simulink model "SMC"  (R2018a)
settings: Solver=FixedStepAuto  StartTime=0.0  StopTime=tsim  FixedStep=ts  RelTol=1e-3
values from neighbouring files (symbols this model uses):
  m = 1    [SMCstart.m]
settings Model: Creator=Chi  LastModifiedBy=Chi

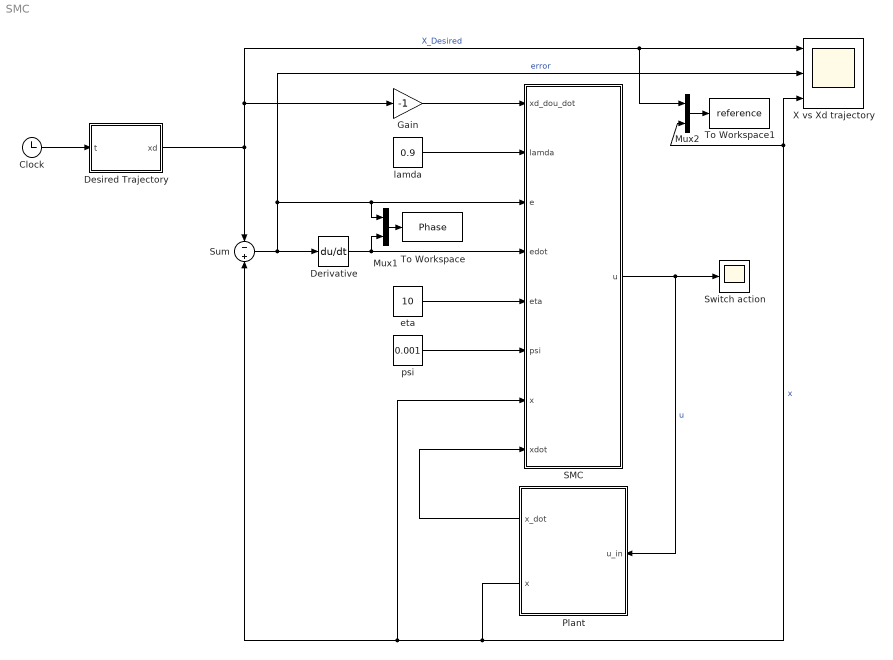
== system SMC ==
  Clock : Clock
  Derivative : Derivative
  Desired Trajectory : MATLAB Function  TreatAsAtomicUnit=on
  Gain : Gain  Gain=-1
  Mux1 : Mux  Inputs=2
  Mux2 : Mux  Inputs=2
  Plant : Subsystem
  SMC : MATLAB Function  TreatAsAtomicUnit=on
  Sum : Sum  Inputs=-+
  Switch action : Scope
  To Workspace : ToWorkspace  VariableName=Phase  SampleTime=-1
  To Workspace1 : ToWorkspace  VariableName=reference  SampleTime=-1
  X vs Xd trajectory : Scope  NumInputPorts=3
  eta : Constant  Value=10
  lamda : Constant  Value=0.9
  psi : Constant  Value=0.001
  wires:
  Clock/1 -> Desired Trajectory/1(t)
  Plant/2(x) -> SMC/7(x), Sum/2, Mux2/2, X vs Xd trajectory/3  "x"
  Desired Trajectory/1(xd) -> Gain/1, X vs Xd trajectory/1, Mux2/1, Sum/1  "X_Desired"
  SMC/1(u) -> Switch action/1, Plant/1(u_in)  "u"
  Sum/1 -> X vs Xd trajectory/2, SMC/3(e), Mux1/1, Derivative/1  "error"
  Derivative/1 -> Mux1/2, SMC/4(edot)
  lamda/1 -> SMC/2(lamda)
  Gain/1 -> SMC/1(xd_dou_dot)
  Plant/1(x_dot) -> SMC/8(xdot)
  eta/1 -> SMC/5(eta)
  Mux1/1 -> To Workspace/1
  psi/1 -> SMC/6(psi)
  Mux2/1 -> To Workspace1/1

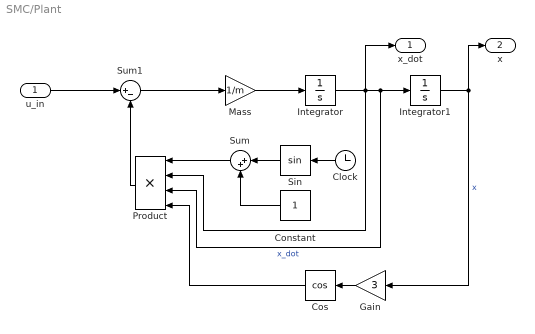
== system SMC/Plant ==
  u_in : Inport
  Clock : Clock
  Constant : Constant
  Cos : Trigonometry  Operator=cos
  Gain : Gain  Gain=3
  Integrator : Integrator
  Integrator1 : Integrator
  Mass : Gain  Gain=1/m
  Product : Product  Inputs=4
  Sin : Trigonometry
  Sum : Sum  Inputs=|++
  Sum1 : Sum  Inputs=|+-
  x_dot : Outport
  x : Outport  Port=2
  wires:
  Sum/1 -> Product/1
  Integrator/1 -> Product/3, Integrator1/1, x_dot/1, Product/2  "x_dot"
  Mass/1 -> Integrator/1
  Constant/1 -> Sum/2
  Sum1/1 -> Mass/1
  Sin/1 -> Sum/1
  Integrator1/1 -> x/1, Gain/1  "x"
  Clock/1 -> Sin/1
  Gain/1 -> Cos/1
  Product/1 -> Sum1/2
  u_in/1 -> Sum1/1
  Cos/1 -> Product/4

== matlab function SMC/SMC ==
  data: u output; xd_dou_dot input; lamda input; e input; edot input; eta input; psi input; x input; xdot input
function u = smc(xd_dou_dot, lamda, e, edot, eta, psi, x, xdot)

    % choose s to satisfy 1. s_dot contains u, 2. s goes to 0, error goes to 0
    s = edot + lamda * e;
    
    %f_hat is our estimation, what's a resaonable guess for our system?
    f_hat = 1.5 * xdot^2 * cos(3*x);
    
    % sliding condition: 1/2 * d(s^2)/dt =< eta * abs(s)
    % we want to make sure the state goes to s = 0
    % choose k = F + eta, F is the max uncertainty, like how good our estimation is
    k = 0.5 * xdot^2 * abs(cos(3*x)) + eta;  
    
    % u_hat would keep s_dot 0 if we knwo everything(knowing that f_hat = f)
    u_hat = - f_hat + xd_dou_dot - lamda * edot;
    
    %k*sign(s) pushing the state back to s = 0
    %u = u_hat - k* sign(s);
    
% Saturation control, this provide a smoother transition
    % thickness of the boundary layer, lower this value means more switching(less tolerance)
     
    
    if (abs(s) > psi)    
        sat_s = sign(s/psi);
    else
        sat_s = s/psi;
    end
    
    u = u_hat - k* sat_s;
    
    %u = 1.5 * xdot^2 * cos(3*x) + xd_dou_dot - lamda * edot - k * sat_s;
   

end

== matlab function SMC/Desired Trajectory ==
  data: t input; xd output
function xd = xdgenerator(t)

xd = sin(pi*t/2);

end
